simulink model "Helicopter_Interface"  (R2022a)
settings: Solver=ode1  StartTime=0.0  StopTime=inf  FixedStep=0.01  MaxStep=0.01  RelTol=1e-3
values from neighbouring files (symbols this model uses):
  A = eval(subs(A_,{x1,x2,x3,x4,x5,x6,F_f,F_b},{0,-5*pi/180,0,0,0,0, u_ap(1)   u_ap(2)}))    [solve.m]
  B = eval(subs(B_,{x1,x2,x3,x4,x5,x6,F_f,F_b},{0,-5*pi/180,0,0,0,0, u_ap(1)   u_ap(2)}))    [solve.m]
  C = [1 0 0 0 0 0 ... (first row only)    [solve.m]
  L = place(A',C',p_beo)'    [Beobachter.m]
  V = -pinv(C*inv(A-B*K)*B)    [Beobachter.m]
undefined symbols (not defined in the file or in its folder): GUIdisplay, K_lqi, u_a, x_init
libraries: vrlib x4, simulink_extras x3
settings Model: Creator=kilia  LastModifiedBy=Lyn
settings SolverCC: AlgebraicLoopSolver=TrustRegion
settings DebuggingCC: UnconnectedInputMsg=warning  UnconnectedOutputMsg=warning  UnconnectedLineMsg=warning
settings RTWCC: DLArmComputeVersion=19.05

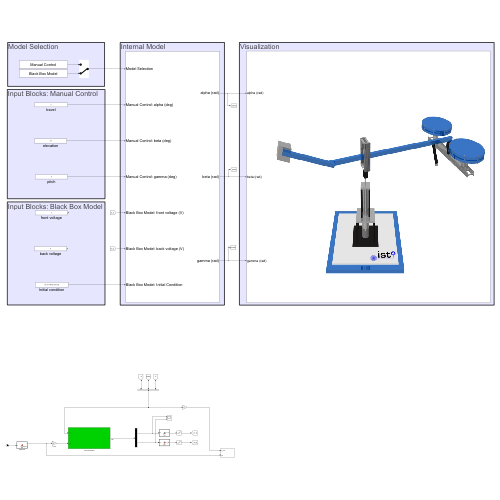
[thumbnail: Simulink's stored preview of the top-level diagram]
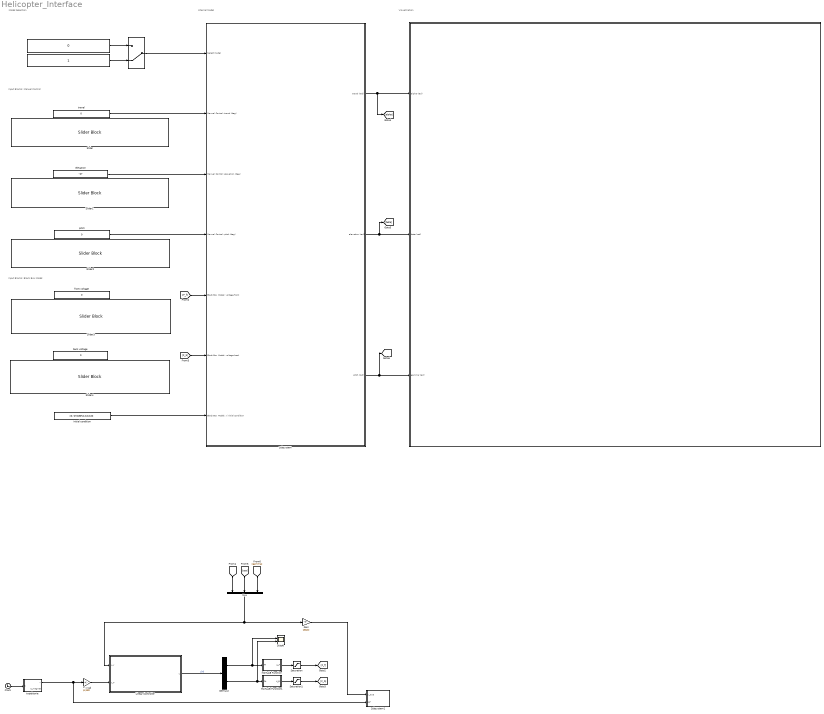
== system Helicopter_Interface ==
  note: Input Blocks: Black Box Model
  note: Internal Model
  note: Visualization
  note: Input Blocks: Manual Control
  note: Model Selection
  "  " : Subsystem
      mask Display: image('$imagefile'); % Use "Edit Image" on toolstrip to change.
  "   " : ManualSwitch  CurrentSetting=0
  "     " : Constant  Value=0
      mask Display: disp('Manual Control');
  "      " : Constant
      mask Display: disp('Black Box Model');
  Clock : Clock
  Demux2 : Demux  Outputs=2
  Gain : Gain  Gain=180/pi
  Initial condition : Constant  Value=[0,-27/180*pi,0,0,0,0]
  Linear Controller : Subsystem
  MATLAB Function : MATLAB Function  TreatAsAtomicUnit=on
  MATLAB Function1 : MATLAB Function  TreatAsAtomicUnit=on
  Mux : Mux  Inputs=3
  Saturation : Saturate  UpperLimit=4  LowerLimit=-4
  Saturation1 : Saturate  UpperLimit=4  LowerLimit=-4
  Scope : Scope  NumInputPorts=2
  Slider : SliderBlock  ScaleMin=-360  ScaleMax=360  TickInterval=90
  Slider1 : SliderBlock  ScaleMin=-27  ScaleMax=30
  Slider2 : SliderBlock  ScaleMin=-90  ScaleMax=90  TickInterval=15
  Slider3 : SliderBlock  ScaleMax=4  TickInterval=0.5
  Slider4 : SliderBlock  ScaleMax=4  TickInterval=0.5
  Subsystem : Subsystem
      mask Display:
      | port_label('input', 1, 'Model Selection');
      | port_label('input', 2, 'Manual Control: alpha (deg)');
      | port_label('input', 3, 'Manual Control: beta (deg)');
      | port_label('input', 4, 'Manual Control: gamma (deg)');
      | port_label('input', 5, 'Black Box Model: front voltage (V)');
      | port_label('input', 6, 'Black Box Model: back voltage (V)');
      | port_label('input', 7, 'Black Box Model: Initial Condition')
      | port_label('output', 1, 'alpha (rad)')
      | port_label('output', 2, 'beta (rad)')
      | port_label('output', 3, 'gamma (rad)')
  Subsystem1 : Subsystem
  back voltage : Constant  Value=0
  elevation : Constant  Value=-27
  front voltage : Constant  Value=0
  pitch : Constant  Value=0
  trajektorie : MATLAB Function  TreatAsAtomicUnit=on
  travel : Constant  Value=0
  °->rad : Gain  Gain=pi/180
  wires:
  "     "/1 -> "   "/1
  "      "/1 -> "   "/2
  "   "/1 -> Subsystem/1(Select model)
  travel/1 -> Subsystem/2(Manual Control: travel (deg))
  elevation/1 -> Subsystem/3(Manual Control: elevation (deg))
  pitch/1 -> Subsystem/4(Manual Control: pitch (deg))
  Initial condition/1 -> Subsystem/7(Black Box Model: x initial condition)
  Subsystem/1(travel (rad)) -> [alpha], "  "/1(alpha (rad))
  Subsystem/2(elevation (rad)) -> [beta], "  "/2(beta (rad))
  Subsystem/3(pitch (rad)) -> [gamma], "  "/3(gamma (rad))
  trajektorie/1(r) -> Subsystem1/2(ref), °->rad/1
  MATLAB Function1/1(U_B) -> Saturation1/1
  °->rad/1 -> Linear Controller/2(y_s)
  MATLAB Function/1(U_F) -> Saturation/1
  Linear Controller/1(u) -> Demux2/1  "u[N]"
  Clock/1 -> trajektorie/1(t)
  Demux2/1 -> Scope/1, MATLAB Function/1(Ff)
  Demux2/2 -> Scope/2, MATLAB Function1/1(Fb)
  Saturation/1 -> [F_f]
  Saturation1/1 -> [F_b]
  [F_f] -> Subsystem/5(Black Box Model: voltage front)
  [F_b] -> Subsystem/6(Black Box Model: voltage back)
  [alpha] -> Mux/1
  [beta] -> Mux/2
  [gamma] -> Mux/3
  Mux/1 -> Linear Controller/1(y_r), Gain/1
  Gain/1 -> Subsystem1/1(y_true)

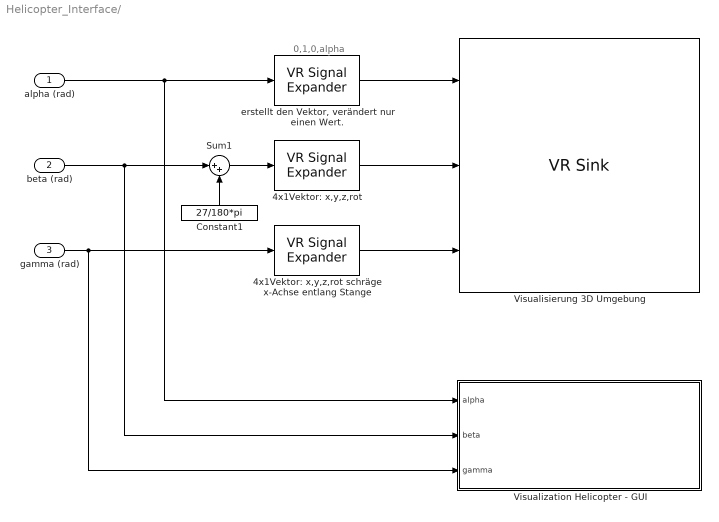
== system Helicopter_Interface/   ==
  note: 0,1,0,alpha
  alpha (rad) : Inport
  beta (rad) : Inport  Port=2
  gamma (rad) : Inport  Port=3
  4x1Vektor: x,y,z,rot : vrlib/VR Signal Expander  outwidth=4  outidx=[4]
  4x1Vektor: x,y,z,rot schräge x-Achse entlang Stange : vrlib/VR Signal Expander  outwidth=4  outidx=[4]
  Constant1 : Constant  Value=27/180*pi
  Sum1 : Sum  Inputs=|++
  Visualisierung 3D Umgebung : vrlib/VR Sink  InstantiateOnLoad=on  SampleTime=-1  ViewEnable=on  RemoteChange=off  RemoteView=off  FieldsWritten=Gelenk_alpha.rotation.4.1.1.double#Gelenk_beta.rotation.4.1.1.double#Gelenk_gamma.rotation.4.1.1.double  WorldFileName=ressources\VrWorld.x3d  AutoView=on  VideoDimensions=[]  AllowVariableSize=off  FigureProperties="{'Position', 'Name', 'Viewpoint', 'CameraBound', 'CameraDirection', 'CameraPosition', 'CameraUpVector', 'ZoomFactor', 'Antialiasing', 'Headlight', 'Lighting', 'NavPanel', 'Sound', 'StatusBar', 'Stereo3D', 'Stereo3DCameraOffset', 'Stereo3DHIT', 'ToolBar', 'Textures', 'Transparency', 'Triad', 'Wireframe', 'NavZones', 'NavMode', 'NavSpeed', 'CaptureFileFormat', 'CaptureFileName', 'Record2DCompressMethod', 'Record2DCompressQuality', 'Record2D', 'Record2DFileName', 'Record2DFPS'; [5.0000000000000000e+00   9.2000000000000000e+01   5.7600000000000000e+02   3.5000000000000000e+02], '', 'seitlich', 'on', [0.0000000000000000e+00   0.0000000000000000e+00  -1.0000000000000000e+00], [0.0000000000000000e+00   0.0000000000000000e+00   0.0000000000000000e+00], [0.0000000000000000e+00   1.0000000000000000e+00   0.0000000000000000e+00], [1.0000000000000000e+00], 'off', 'on', 'on', 'halfbar', 'on', 'on', 'off', [1.0000000149011612e-01], [0.0000000000000000e+00], 'on', 'on', 'on', 'none', 'off', 'off', 'fly', 'normal', 'tif', '%f_anim_%n.tif', 'auto', [7.5000000000000000e+01], 'off', '%f_anim_%n.avi', 'auto'}"
  Visualization Helicopter - GUI : Subsystem  LoadFcn=GUIdisplay([], [], [], 'LoadBlock', [], [])  StartFcn=GUIdisplay([], [], [], 'Start', [], 'ressources/VrWorld.x3d')  StopFcn=GUIdisplay([], [], [], 'Stop', [], [])  mask(Grafische Benutzeroberfläche){y1range=[-100 470], y2range=[-32 35], y3range=[-95 95], worldfile=ressources/VrWorld.x3d}
      mask prompts: y1range "Alpha range:"; y2range "Beta range:"; y3range "Gamma range:"; worldfile "VRML World Datei:"
      mask help:
      | Anzeige der grafischen Benutzeroberfläche.
      |
      | 2 VR Kameraperspektiven,
      | 3 Plots für die 3 Winkel.
      settings: CopyFcn=GUIdisplay([], [], [], 'CopyBlock', [], [])  DeleteFcn=GUIdisplay([], [], [], 'DeleteBlock', [], [])  NameChangeFcn=GUIdisplay([], [], [], 'NameChange', [], [])
      mask Display:
      | port_label('input',1,'alpha');
      | port_label('input',2,'beta');
      | port_label('input',3,'gamma');
      | image('ressources/GUImask.png');
  "erstellt den Vektor, verändert nur einen Wert." : vrlib/VR Signal Expander  outwidth=4  outidx=[4]
  wires:
  alpha (rad)/1 -> "erstellt den Vektor, verändert nur einen Wert."/1, Visualization Helicopter - GUI/1(alpha)
  "erstellt den Vektor, verändert nur einen Wert."/1 -> Visualisierung 3D Umgebung/1
  4x1Vektor: x,y,z,rot/1 -> Visualisierung 3D Umgebung/2
  4x1Vektor: x,y,z,rot schräge x-Achse entlang Stange/1 -> Visualisierung 3D Umgebung/3
  Constant1/1 -> Sum1/2
  beta (rad)/1 -> Sum1/1, Visualization Helicopter - GUI/2(beta)
  gamma (rad)/1 -> 4x1Vektor: x,y,z,rot schräge x-Achse entlang Stange/1, Visualization Helicopter - GUI/3(gamma)
  Sum1/1 -> 4x1Vektor: x,y,z,rot/1

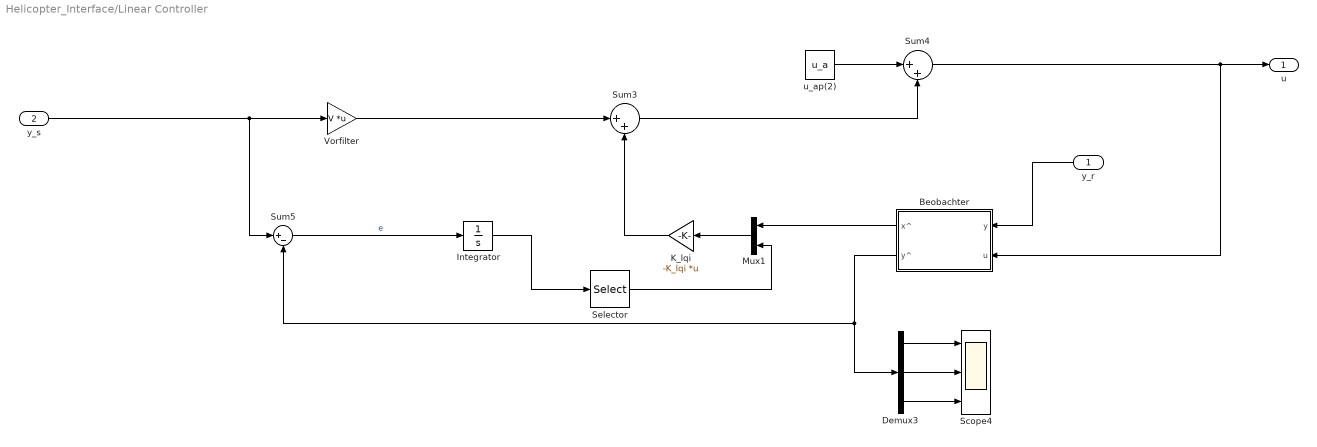
== system Helicopter_Interface/Linear Controller ==
  y_r : Inport
  y_s : Inport  Port=2
  Beobachter : Subsystem
  Demux3 : Demux  Outputs=3
  Integrator : Integrator
  K_lqi : Gain  Gain=-K_lqi  Multiplication=Matrix(K*u) (u vector)
  Mux1 : Mux  Inputs=2
  Scope4 : Scope  NumInputPorts=3
  Selector : Selector  InputPortWidth=3  IndexOptions=Index vector (dialog)  Indices=[1 2]  OutputSizes=1
  Sum3 : Sum  Inputs=|++
  Sum4 : Sum  Inputs=|++
  Sum5 : Sum  Inputs=|+-
  Vorfilter : Gain  Gain=V  Multiplication=Matrix(K*u) (u vector)
  u_ap(2) : Constant  Value=u_a  VectorParams1D=off
  u : Outport
  wires:
  u_ap(2)/1 -> Sum4/1
  Sum3/1 -> Sum4/2
  Sum5/1 -> Integrator/1  "e"
  Beobachter/1(x^) -> Mux1/1
  Demux3/2 -> Scope4/2
  K_lqi/1 -> Sum3/2
  Sum4/1 -> Beobachter/2(u), u/1
  Demux3/1 -> Scope4/1
  Mux1/1 -> K_lqi/1
  Vorfilter/1 -> Sum3/1
  y_s/1 -> Vorfilter/1, Sum5/1
  Beobachter/2(y^) -> Sum5/2, Demux3/1
  Integrator/1 -> Selector/1
  Selector/1 -> Mux1/2
  Demux3/3 -> Scope4/3
  y_r/1 -> Beobachter/1(y)

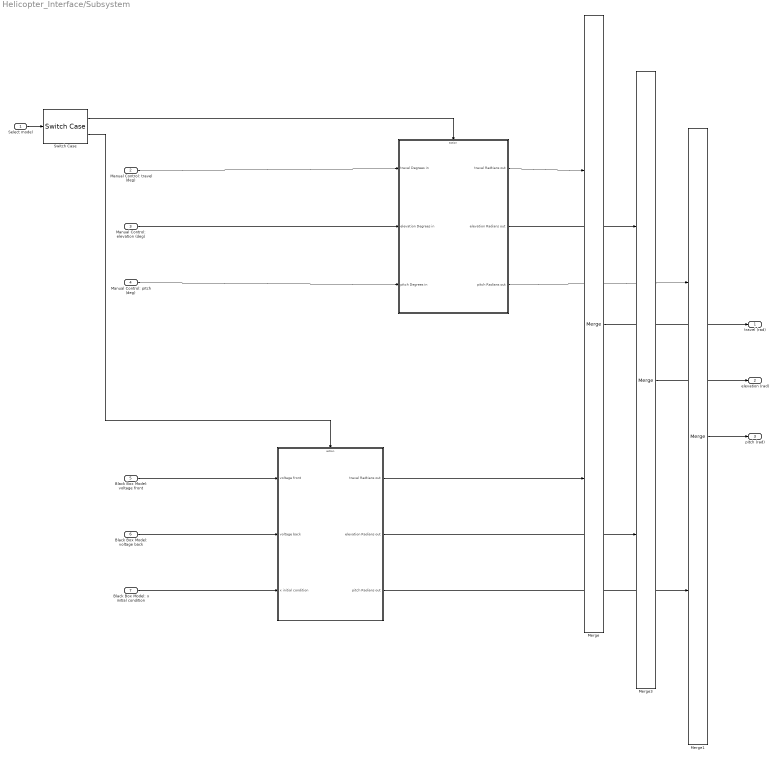
== system Helicopter_Interface/Subsystem ==
  Select model : Inport
  Manual Control: travel (deg) : Inport  Port=2
  Manual Control: elevation (deg) : Inport  Port=3
  Manual Control: pitch (deg) : Inport  Port=4
  Black Box Model: voltage front : Inport  Port=5
  Black Box Model: voltage back : Inport  Port=6
  Black Box Model: x initial condition : Inport  Port=7
  " " : Subsystem  TreatAsAtomicUnit=on
      mask Display: disp('Manual Control');
  "  " : Subsystem  TreatAsAtomicUnit=on
      mask Display: disp('Black Box Model');
  Merge : Merge
  Merge1 : Merge
  Merge3 : Merge
  Switch Case : SwitchCase  CaseConditions={0,1}  ShowDefaultCase=off
  travel (rad) : Outport
  elevation (rad) : Outport  Port=2
  pitch (rad) : Outport  Port=3
  wires:
  "  "/1(travel Radtians out) -> Merge/2
  " "/1(travel Radtians out) -> Merge/1
  "  "/2(elevation Radians out) -> Merge3/2
  Black Box Model: x initial condition/1 -> "  "/3(x initial condition)
  "  "/3(pitch Radians out) -> Merge1/2
  " "/3(pitch Radians out) -> Merge1/1
  " "/2(elevation Radians out) -> Merge3/1
  Switch Case/1 -> " "/Action
  Manual Control: elevation (deg)/1 -> " "/2(elevation Degrees in)
  Switch Case/2 -> "  "/Action
  Merge3/1 -> elevation (rad)/1
  Merge1/1 -> pitch (rad)/1
  Merge/1 -> travel (rad)/1
  Black Box Model: voltage back/1 -> "  "/2(voltage back)
  Manual Control: pitch (deg)/1 -> " "/3(pitch Degrees in)
  Black Box Model: voltage front/1 -> "  "/1(voltage front)
  Manual Control: travel (deg)/1 -> " "/1(travel Degrees in)
  Select model/1 -> Switch Case/1

== system Helicopter_Interface/Subsystem1 ==
  y_true : Inport
  ref : Inport  Port=2
  Demux : Demux  Outputs=3
  Demux1 : Demux  Outputs=3
  Scope : Subsystem
  wires:
  Demux/2 -> Scope/2(beta_r[°])  "beta_r[°]"
  Demux1/1 -> Scope/4(alpha_s[°])
  Demux1/3 -> Scope/6(gamma_s[°])
  Demux/3 -> Scope/3(gamma_r[°])
  Demux1/2 -> Scope/5(beta_s[°])
  Demux/1 -> Scope/1(alpha_r[°])  "alpha_r[°]"
  y_true/1 -> Demux/1
  ref/1 -> Demux1/1

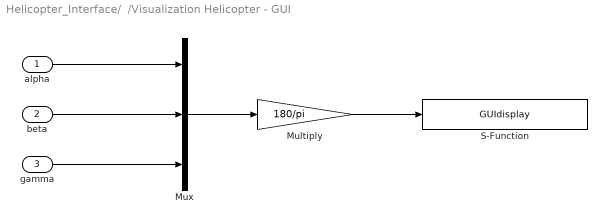
== system Helicopter_Interface/  /Visualization Helicopter - GUI ==
  alpha : Inport
  beta : Inport  Port=2
  gamma : Inport  Port=3
  Multiply : Gain  Gain=180/pi
  Mux : Mux  Inputs=3
  S-Function : S-Function  FunctionName=GUIdisplay  Parameters=[y1range y2range y3range], worldfile  SFunctionDeploymentMode=off  EnableBusSupport=off
  wires:
  Multiply/1 -> S-Function/1
  alpha/1 -> Mux/1
  gamma/1 -> Mux/3
  Mux/1 -> Multiply/1
  beta/1 -> Mux/2

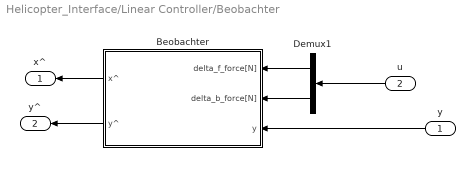
== system Helicopter_Interface/Linear Controller/Beobachter ==
  y : Inport
  u : Inport  Port=2
  Beobachter : Subsystem
  Demux1 : Demux  Outputs=2
  x^ : Outport
  y^ : Outport  Port=2
  wires:
  u/1 -> Demux1/1
  Demux1/1 -> Beobachter/1(delta_f_force[N])
  Demux1/2 -> Beobachter/2(delta_b_force[N])
  Beobachter/1(x^) -> x^/1
  y/1 -> Beobachter/3(y)
  Beobachter/2(y^) -> y^/1

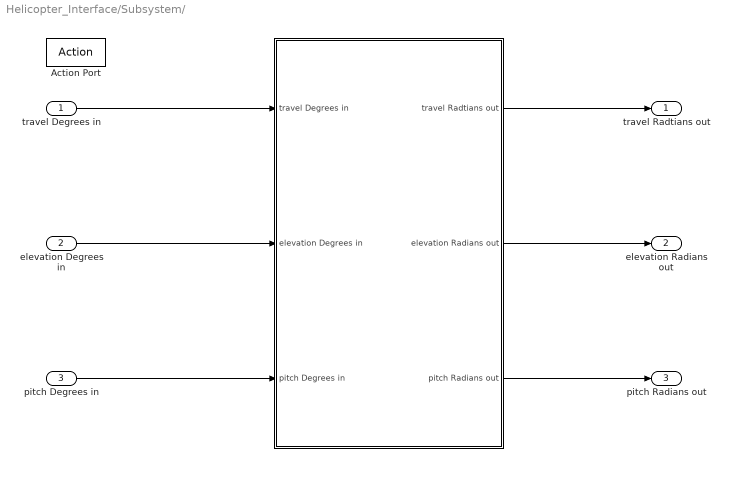
== system Helicopter_Interface/Subsystem/  ==
  travel Degrees in : Inport
  elevation Degrees in : Inport  Port=2
  pitch Degrees in : Inport  Port=3
  Action Port : ActionPort  ActionPortLabel=case [ 0 ]:
  " " : Subsystem
  travel Radtians out : Outport
  elevation Radians out : Outport  Port=2
  pitch Radians out : Outport  Port=3
  wires:
  " "/2(elevation Radians out) -> elevation Radians out/1
  " "/1(travel Radtians out) -> travel Radtians out/1
  " "/3(pitch Radians out) -> pitch Radians out/1
  travel Degrees in/1 -> " "/1(travel Degrees in)
  elevation Degrees in/1 -> " "/2(elevation Degrees in)
  pitch Degrees in/1 -> " "/3(pitch Degrees in)

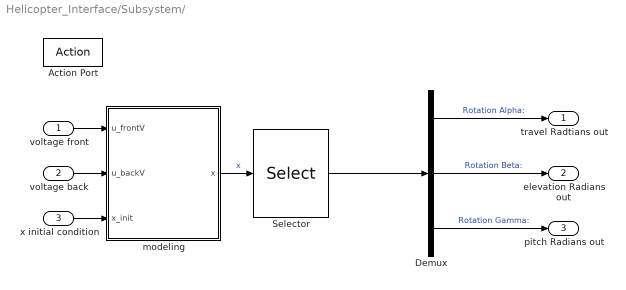
== system Helicopter_Interface/Subsystem/   ==
  voltage front : Inport
  voltage back : Inport  Port=2
  x initial condition : Inport  Port=3
  Action Port : ActionPort  ActionPortLabel=case [ 1 ]:
  Demux : Demux  Outputs=3
  Selector : Selector  InputPortWidth=6  IndexOptions=Index vector (dialog)  Indices=[1 2 3]  OutputSizes=1
  modeling : Subsystem
  travel Radtians out : Outport
  elevation Radians out : Outport  Port=2
  pitch Radians out : Outport  Port=3
  wires:
  Selector/1 -> Demux/1
  Demux/1 -> travel Radtians out/1  "Rotation Alpha:"
  modeling/1(x) -> Selector/1  "x"
  Demux/3 -> pitch Radians out/1  "Rotation Gamma:"
  Demux/2 -> elevation Radians out/1  "Rotation Beta:"
  voltage front/1 -> modeling/1(u_frontV)
  voltage back/1 -> modeling/2(u_backV)
  x initial condition/1 -> modeling/3(x_init)

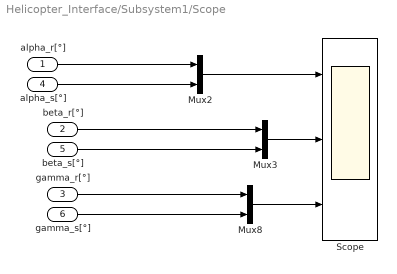
== system Helicopter_Interface/Subsystem1/Scope ==
  alpha_r[°] : Inport
  beta_r[°] : Inport  Port=2
  gamma_r[°] : Inport  Port=3
  alpha_s[°] : Inport  Port=4
  beta_s[°] : Inport  Port=5
  gamma_s[°] : Inport  Port=6
  Mux2 : Mux  Inputs=2
  Mux3 : Mux  Inputs=2
  Mux8 : Mux  Inputs=2
  Scope : Scope  NumInputPorts=3
  wires:
  Mux8/1 -> Scope/3
  Mux2/1 -> Scope/1
  Mux3/1 -> Scope/2
  gamma_r[°]/1 -> Mux8/1
  beta_r[°]/1 -> Mux3/1
  alpha_s[°]/1 -> Mux2/2
  alpha_r[°]/1 -> Mux2/1
  beta_s[°]/1 -> Mux3/2
  gamma_s[°]/1 -> Mux8/2

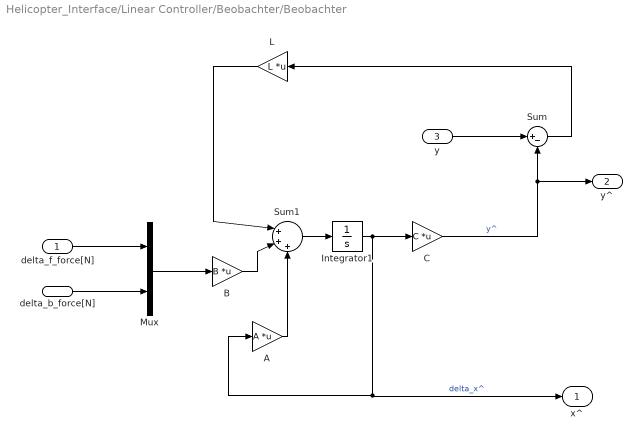
== system Helicopter_Interface/Linear Controller/Beobachter/Beobachter ==
  delta_f_force[N] : Inport
  delta_b_force[N] : Inport  Port=2
  y : Inport  Port=3
  A : Gain  Gain=A  Multiplication=Matrix(K*u) (u vector)
  B : Gain  Gain=B  Multiplication=Matrix(K*u) (u vector)
  C : Gain  Gain=C  Multiplication=Matrix(K*u) (u vector)
  Integrator1 : Integrator  InitialCondition=[0;-27*pi/180;0;0;0;0]
  L : Gain  Gain=L  Multiplication=Matrix(K*u) (u vector)
  Mux : Mux  Inputs=2
  Sum : Sum  Inputs=|+-
  Sum1 : Sum  Inputs=|+++
  x^ : Outport
  y^ : Outport  Port=2
  wires:
  Sum1/1 -> Integrator1/1
  Integrator1/1 -> C/1, x^/1, A/1  "delta_x^"
  B/1 -> Sum1/2
  L/1 -> Sum1/1
  Sum/1 -> L/1
  Mux/1 -> B/1
  A/1 -> Sum1/3
  C/1 -> y^/1, Sum/2  "y^"
  delta_f_force[N]/1 -> Mux/1
  delta_b_force[N]/1 -> Mux/2
  y/1 -> Sum/1

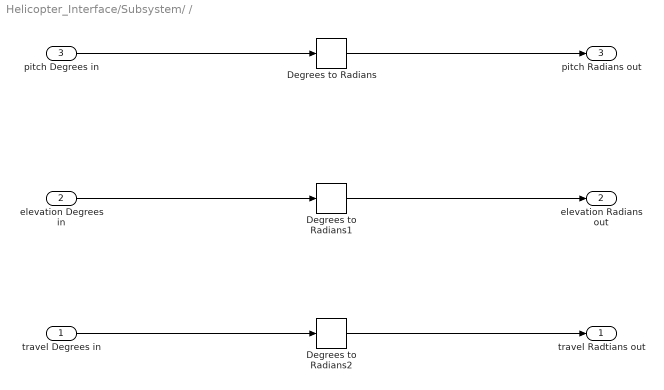
== system Helicopter_Interface/Subsystem/ /  ==
  travel Degrees in : Inport
  elevation Degrees in : Inport  Port=2
  pitch Degrees in : Inport  Port=3
  Degrees to Radians : simulink_extras/Transformations/Degrees to Radians
  Degrees to Radians1 : simulink_extras/Transformations/Degrees to Radians
  Degrees to Radians2 : simulink_extras/Transformations/Degrees to Radians
  travel Radtians out : Outport
  elevation Radians out : Outport  Port=2
  pitch Radians out : Outport  Port=3
  wires:
  pitch Degrees in/1 -> Degrees to Radians/1
  Degrees to Radians/1 -> pitch Radians out/1
  Degrees to Radians2/1 -> travel Radtians out/1
  Degrees to Radians1/1 -> elevation Radians out/1
  travel Degrees in/1 -> Degrees to Radians2/1
  elevation Degrees in/1 -> Degrees to Radians1/1

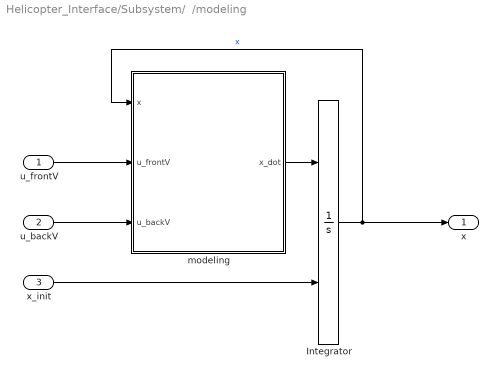
== system Helicopter_Interface/Subsystem/  /modeling ==
  u_frontV : Inport
  u_backV : Inport  Port=2
  x_init : Inport  Port=3
  Integrator : Integrator  InitialConditionSource=external  InitialCondition=x_init
  modeling : MATLAB Function  TreatAsAtomicUnit=on
  x : Outport
  wires:
  modeling/1(x_dot) -> Integrator/1
  Integrator/1 -> x/1, modeling/1(x)  "x"
  x_init/1 -> Integrator/2
  u_backV/1 -> modeling/3(u_backV)
  u_frontV/1 -> modeling/2(u_frontV)

== matlab function Helicopter_Interface/MATLAB Function ==
  data: Ff input; U_F output
function U_F = fcn(Ff)
    U_F= sqrt(20*abs(Ff));
end

== matlab function Helicopter_Interface/Subsystem/  /modeling/modeling ==
  data: x input; x_dot output; u_frontV input; u_backV input
function x_dot = modeling(x,u_frontV,u_backV)
    if u_frontV > 4
        u_frontV = 4;
    elseif u_frontV < -4
        u_frontV = -4;
    end
    if u_backV > 4
        u_backV = 4;
    elseif u_backV < -4
        u_backV = -4;
    end
    t2 = cos(x(2));
    t3 = cos(x(3));
    t4 = sin(x(2));
    t5 = sin(x(3));
    t6 = x(4).^2;
    t7 = x(2).*2.0;
    t8 = x(5).^2;
    t9 = x(3).*2.0;
    t10 = x(6).^2;
    t11 = u_backV.^2;
    t12 = u_frontV.^2;
    t48 = x(4).*x(5).*2.03058268355089e-1;
    t13 = cos(t7);
    t14 = t2.^2;
    t15 = t3.^2;
    t16 = t3.^3;
    t18 = sin(t7);
    t19 = t4.^2;
    t20 = sin(t9);
    t21 = t5.^2;
    t23 = t2.*t8.*1.635155998723047e-2;
    t25 = t11.*9.174434079640917e-3;
    t26 = t12.*9.174434079640917e-3;
    t27 = x(4).*x(5).*t2.*7.452385e-2;
    t28 = t4.*t8.*4.862799017853676e-4;
    t29 = x(4).*x(6).*t2.*7.452385e-2;
    t33 = t3.*t11.*3.385495392768902e-2;
    t34 = t3.*t12.*3.385495392768902e-2;
    t35 = t5.*t11.*2.946156295997365e-3;
    t36 = t5.*t12.*2.946156295997365e-3;
    t41 = t2.*t5.*t11.*3.385495392768902e-2;
    t42 = t2.*t5.*t12.*3.385495392768902e-2;
    t43 = t4.*t12.*(-9.174434079640917e-3);
    t44 = t4.*t5.*t11.*4.600138777960798e-3;
    t45 = t4.*t5.*t12.*4.600138777960798e-3;
    t46 = t2.*t3.*t11.*2.946156295997365e-3;
    t47 = t2.*t3.*t12.*2.946156295997365e-3;
    t49 = t6.*1.015291341775445e-1;
    t50 = -t48;
    t52 = x(4).*x(5).*t3.*2.774580000000001e-3;
    t53 = x(4).*x(6).*t5.*3.770040000000002e-4;
    t54 = x(5).*x(6).*t5.*3.770040000000002e-4;
    t55 = t3.*t6.*1.387290000000001e-3;
    t57 = t3.*t10.*1.387290000000001e-3;
    t58 = t5.*t6.*1.885020000000001e-4;
    t59 = t5.*t8.*1.885020000000001e-4;
    t64 = x(4).*x(6).*t3.*t4.*2.774580000000001e-3;
    t65 = x(4).*x(5).*t2.*t3.*3.770040000000002e-4;
    t66 = x(4).*x(6).*t2.*t3.*3.770040000000002e-4;
    t68 = x(4).*x(5).*t2.*t3.*t4.*7.540080000000003e-4;
    t69 = t2.*t5.*t8.*1.387290000000001e-3;
    t70 = x(4).*x(5).*t3.*t4.*(-2.774580000000001e-3);
    t71 = t2.*t5.*t10.*1.387290000000001e-3;
    t74 = t4.*t5.*t10.*1.885020000000001e-4;
    t75 = x(4).*x(6).*t2.*t4.*t5.*2.774580000000001e-3;
    t80 = t2.*t4.*t5.*t6.*1.387290000000001e-3;
    t82 = t2.*t3.*t4.*t6.*3.770040000000002e-4;
    t91 = t2.*8.248718165204683e-1;
    t92 = t2.*t5.*4.155516000000001e-2;
    t93 = t3.*t4.*4.155516000000001e-2;
    t94 = t4.*1.324177010693453;
    t95 = t2.*6.321561677527197e+77;
    t97 = t3.*1.225248066969451e+78;
    t98 = t2.*t5.*2.450496133938901e+77;
    t99 = t4.*2.125676891098147e+79;
    t100 = t2.*t5.*7.094850583348527e+78;
    t101 = t3.*t5.*1.100101830038337e+78;
    t102 = x(5).*x(6).*t2.*2.73147057186082e-3;
    t103 = t3.*t4.*t5.*8.800814640306698e+75;
    t105 = t5.*3.48026202342401e+81;
    t106 = t2.*t3.*t5.*6.477004033034705e+76;
    t107 = t4.*t5.*2.385701619337445e+80;
    t112 = t2.*t4.*7.901952096908996e+79;
    t113 = t3.*t4.*2.509206552712654e+81;
    t114 = t4.*4.827997583224782e+83;
    t119 = t2.*t4.*t5.*3.063120167423627e+79;
    t132 = t2.*t3.*t4.*9.50424515204181e+79;
    t133 = t2.*t3.*1.733947310723218e+82;
    t146 = t2.*t3.*t4.*t5.*7.946775555990462e+78;
    t158 = t3.*t4.*t5.*t8.*3.589618971406959e-2;
    t171 = t3.*9.694963676602881e+122;
    t174 = t2.*t4.*3.434970881571123e+121;
    t187 = t2.*t4.*t5.*1.331535353899349e+121;
    t193 = t2.*t3.*t4.*t5.*3.505212574967064e+120;
    t223 = t2.*t3.*t4.*7.122357460232167e+123;
    t17 = t15.^2;
    t22 = t20.^2;
    t24 = -t23;
    t30 = -t26;
    t31 = -t28;
    t32 = -t29;
    t37 = -t33;
    t38 = -t34;
    t39 = t4.*t25;
    t40 = t4.*t26;
    t51 = x(4).*x(5).*t14.*4.061165367101779e-1;
    t56 = -t52;
    t60 = -t53;
    t61 = -t54;
    t62 = t6.*t14.*2.03058268355089e-1;
    t63 = t4.*t52;
    t72 = -t66;
    t73 = t4.*t59;
    t76 = -t71;
    t77 = -t74;
    t78 = x(4).*x(5).*t3.*t14.*5.549160000000002e-3;
    t79 = t14.*t53;
    t81 = -t75;
    t83 = t3.*t6.*t14.*2.774580000000001e-3;
    t84 = t14.*t58;
    t85 = -t82;
    t86 = x(4).*x(5).*t18.*1.086802113522521;
    t88 = t5.*t6.*t14.*(-1.885020000000001e-4);
    t89 = t6.*t18.*5.434010567612607e-1;
    t96 = -t95;
    t104 = -t100;
    t108 = t2.*t15.*5.500509150191686e+78;
    t109 = t3.*t14.*2.837940233339411e+78;
    t110 = t2.*t21.*2.750254575095843e+78;
    t111 = t15.*1.166611947319722e+80;
    t116 = t3.*t19.*1.296656147304016e+79;
    t117 = t4.*t21.*2.024063760323345e+79;
    t118 = t19.*2.657096113872683e+81;
    t120 = t2.*t20.*2.333223894639443e+79;
    t121 = -t112;
    t122 = t13.*t101;
    t123 = t14.*t101;
    t124 = t19.*t101;
    t125 = t2.*t16.*5.237273874528027e+80;
    t126 = t4.*t16.*7.116295798977013e+79;
    t127 = t5.*t15.*1.047454774905605e+80;
    t128 = t5.*t18.*5.925262666227655e+80;
    t130 = t5.*t19.*2.254318774901658e+80;
    t131 = x(5).*x(6).*t20.*3.589618971406959e-2;
    t135 = t3.*t5.*t13.*-1.100101830038337e+78;
    t136 = t3.*t5.*t18.*8.096255041293381e+78;
    t137 = t3.*t5.*t19.*-1.100101830038337e+78;
    t139 = x(4).*x(5).*t2.*t15.*7.179237942813918e-2;
    t140 = x(4).*x(6).*t2.*t15.*7.179237942813918e-2;
    t141 = x(5).*x(6).*t2.*t15.*7.179237942813918e-2;
    t142 = t5.*t13.*3.171300553775711e+81;
    t145 = t8.*t20.*1.79480948570348e-2;
    t147 = t2.*t5.*t20.*2.618636937264013e+80;
    t150 = -t146;
    t151 = t4.*t15.*1.458190194407001e+82;
    t152 = t2.*t3.*t4.*t20.*1.423259159795403e+79;
    t154 = x(4).*x(6).*t3.*t5.*t14.*7.179237942813918e-2;
    t156 = t2.*t4.*t20.*2.916529868299304e+81;
    t160 = x(4).*x(5).*t2.*t4.*t15.*(-7.179237942813918e-2);
    t164 = t3.*t14.*t20.*1.047454774905605e+80;
    t165 = -t158;
    t166 = t2.*t4.*t6.*t15.*3.589618971406959e-2;
    t167 = t3.*t5.*t6.*t14.*3.589618971406959e-2;
    t169 = t14.*5.107638978270105e+119;
    t170 = t3.*t21.*2.028614954006237e+118;
    t172 = t5.*t14.*3.959859986591955e+119;
    t173 = t21.*6.417689155495646e+121;
    t175 = -t171;
    t177 = t15.*1.641540254081147e+122;
    t178 = t14.*t16.*4.057229908012474e+118;
    t179 = t14.*t21.*7.675019309373171e+118;
    t181 = -t174;
    t182 = t3.*t5.*t14.*1.046646381040499e+119;
    t183 = t3.*t5.*t19.*4.782131942337327e+119;
    t184 = t3.*t13.*4.138462702746391e+121;
    t191 = t3.*t14.*t21.*4.057229908012474e+118;
    t192 = t3.*t19.*t21.*4.057229908012474e+118;
    t195 = t15.*t21.*1.931532483628991e+120;
    t196 = t19.*t21.*4.157019516732514e+120;
    t197 = t2.*t3.*t4.*t21.*2.93081009208969e+119;
    t198 = t2.*t4.*t15.*3.7016311010743e+121;
    t200 = t3.*t18.*3.643855631716766e+123;
    t201 = t3.*t19.*9.992258694036609e+122;
    t202 = t3.*t13.*t21.*-2.028614954006237e+118;
    t203 = t18.*2.606256753239576e+125;
    t204 = t19.*9.973487007685766e+124;
    t205 = t3.*t18.*t21.*1.492969432442792e+119;
    t207 = t13.*t16.*2.923087810085905e+121;
    t209 = t13.*t21.*5.847956572177934e+121;
    t210 = t14.*t20.*3.770354832305701e+121;
    t211 = t16.*t19.*2.923012902287755e+121;
    t212 = t18.*t21.*1.09263307476776e+121;
    t215 = t2.*t4.*t16.*2.151150995944596e+122;
    t217 = t13.*1.394912588759959e+126;
    t220 = t14.*t15.*1.27897667213932e+122;
    t221 = t16.*t18.*1.075630626745094e+122;
    t225 = t2.*t4.*t20.*1.267812693620274e+123;
    t227 = t5.*t14.*t20.*1.461543905042952e+121;
    t228 = t13.*t15.*3.940256742008736e+123;
    t230 = t15.*t19.*2.992314274899525e+123;
    t231 = t2.*t3.*t4.*t5.*t20.*5.249050108182602e+119;
    t233 = t3.*t5.*t14.*t20.*3.863064967257982e+120;
    t237 = t15.*t18.*7.870897512302404e+123;
    t67 = -t62;
    t87 = -t83;
    t90 = -t86;
    t115 = -t109;
    t129 = -t117;
    t134 = -t120;
    t138 = -t125;
    t143 = -t126;
    t144 = -t130;
    t148 = -t139;
    t149 = -t145;
    t153 = t4.*t139;
    t155 = -t147;
    t157 = -t151;
    t159 = -t152;
    t161 = -t154;
    t162 = -t156;
    t163 = t13.*t127;
    t168 = -t164;
    t176 = -t172;
    t180 = t17.*t19.*7.132297093561092e+118;
    t185 = t17.*1.391599486765761e+123;
    t188 = t2.*t4.*t17.*1.04981002163652e+120;
    t189 = -t182;
    t190 = t13.*t170;
    t194 = t14.*t17.*3.863064967257982e+120;
    t206 = -t192;
    t213 = -t196;
    t214 = -t197;
    t216 = -t200;
    t218 = -t203;
    t219 = -t207;
    t222 = -t211;
    t224 = -t215;
    t226 = -t217;
    t232 = -t225;
    t234 = -t227;
    t235 = -t228;
    t236 = -t230;
    t238 = -t231;
    t239 = t13.*t195;
    t240 = -t233;
    t241 = t14.*t22.*6.957997433828807e+122;
    t186 = -t180;
    t199 = -t188;
    t208 = -t194;
    t229 = t13.*t185;
    t242 = t96+t98+t99+t103+t106+t134;
    t243 = t25+t27+t30+t58+t59+t65+t70+t80+t88+t92+t148+t149+t167;
    t244 = t104+t107+t108+t110+t113+t114+t129+t133+t138+t143+t155+t157;
    t245 = t32+t35+t36+t37+t38+t49+t55+t57+t61+t64+t67+t72+t85+t87+t89+t91+t93+t94+t131+t140+t166;
    t246 = t24+t31+t39+t41+t42+t43+t44+t45+t46+t47+t50+t51+t56+t60+t68+t69+t73+t76+t77+t78+t79+t81+t90+t102+t141+t160+t161+t165;
    t247 = t101+t105+t115+t116+t118+t119+t121+t123+t127+t128+t132+t135+t136+t137+t142+t144+t150+t159+t162+t163+t168;
    t248 = t169+t170+t173+t175+t176+t177+t178+t179+t181+t183+t184+t185+t186+t187+t189+t191+t193+t195+t198+t199+t201+t202+t204+t205+t206+t208+t209+t210+t212+t213+t214+t216+t218+t219+t220+t221+t222+t223+t224+t226+t229+t232+t234+t235+t236+t237+t238+t239+t240+t241-1.530810853886889e+126;
    t249 = 1.0./t248;
    x_dot = [x(4);x(5);x(6);t242.*t245.*t249.*1.661534994731145e+45-t243.*t244.*t249.*5.316911983139663e+42-t246.*t249.*(t21.*1.619251008258676e+77-t97+t111-3.862398066579826e+81).*6.646139978924579e+44;t245.*t249.*(t13.*3.532063820998669e+81+t18.*6.599313290687543e+80-t19.*2.510767317953594e+80+t97+t111-t3.*t13.*1.225248066969451e+78+t3.*t18.*9.017275099606632e+78-t3.*t19.*2.450496133938901e+78-t14.*t15.*3.238502016517352e+77-t15.*t19.*5.979179412116765e+75+t13.*t111-t2.*t3.*t4.*1.803455019921326e+79-t2.*t4.*t15.*8.800814640306698e+76+3.876172369060467e+81).*3.32306998946229e+44+t242.*t246.*t249.*1.661534994731145e+45-t243.*t247.*t249.*1.329227995784916e+43;t244.*t246.*t249.*-5.316911983139663e+42-t245.*t247.*t249.*1.329227995784916e+43-t243.*t249.*(t3.*-4.95652853788659e+85-t13.*7.131459471819949e+88+t14.*2.611269026011294e+82+t15.*8.392337905379119e+84+t17.*7.114521311831996e+85-t18.*1.332442947224953e+88+t19.*2.952550677741535e+85-t2.*t4.*1.756121195420763e+84+t3.*t13.*2.115779818612926e+84-t5.*t14.*2.024469578668458e+82-t3.*t18.*1.862913057645561e+86-t5.*t19.*5.009973400608635e+84-t13.*t15.*2.014447463635022e+86-t13.*t16.*1.494422117785173e+84+t13.*t17.*7.114521311831996e+85+t15.*t18.*4.02397878319616e+86+t14.*t20.*1.927585491566282e+84+t16.*t18.*5.499137568254428e+84+t14.*t21.*3.923836489201627e+81+t14.*t22.*3.557260655915998e+85+t19.*t21.*2.125266948339513e+83+t2.*t4.*t5.*8.297363395849275e+83-t2.*t4.*t20.*6.48166409513115e+85-t2.*t4.*t21.*5.775534607701271e+82-t5.*t14.*t20.*7.472110588925864e+83+t2.*t4.*t5.*t20.*5.499137568254428e+84-7.826236318665165e+88).*5.063725698228251e+38];
end

== matlab function Helicopter_Interface/MATLAB Function1 ==
  data: Fb input; U_B output
function U_B = fcn(Fb)
    U_B= sqrt(20*abs(Fb));
end

== matlab function Helicopter_Interface/trajektorie ==
  data: t input; r output; U_magnet output
function [r, U_magnet] = fcn(t)
beta = -27;
if t <= 10
    a0 = five_times_plan(0, -27, 0, 0, 10, -5, 0, 0);
    alpha = 0;
    beta = a0(1)+a0(2)*t+a0(3)*t^2+a0(4)*t^3+a0(5)*t^4+a0(6)*t^5;
    U_magnet = 0;
elseif t > 10 && t <= 18
    a0 = five_times_plan(10, 0, 0, 0, 18, 90, 0, 0);
    alpha = a0(1)+a0(2)*t+a0(3)*t^2+a0(4)*t^3+a0(5)*t^4+a0(6)*t^5;
    beta = -5;
    U_magnet = 0;
elseif t > 18 &&t <= 26
    a0 = five_times_plan(18, -5, 0, 0, 26, -22, 0, 0);
    alpha = 90;
    beta = a0(1)+a0(2)*t+a0(3)*t^2+a0(4)*t^3+a0(5)*t^4+a0(6)*t^5;
    U_magnet = 1;
elseif t > 26 && t <= 30
    alpha = 90;
    beta = -22;
    U_magnet = 0;
elseif t > 30 && t <= 38
    a0 = five_times_plan(30, -22, 0, 0, 38, -5, 0, 0);
    alpha = 90;
    beta = a0(1)+a0(2)*t+a0(3)*t^2+a0(4)*t^3+a0(5)*t^4+a0(6)*t^5;
    U_magnet = 0;
elseif t > 38 && t <= 62
    a0 = five_times_plan(38, 90, 0, 0,62, 450, 0, 0);
    alpha = a0(1)+a0(2)*t+a0(3)*t^2+a0(4)*t^3+a0(5)*t^4+a0(6)*t^5;
    beta = -5;
    U_magnet = 0;
elseif t > 62 && t <= 70
    a0 = five_times_plan(62, -5, 0, 0, 70, -22, 0, 0); 
    alpha = 450;
    beta = a0(1)+a0(2)*t+a0(3)*t^2+a0(4)*t^3+a0(5)*t^4+a0(6)*t^5;
    U_magnet = 1;
elseif t > 70 && t <= 74
    alpha = 450;
    beta = -22;
    U_magnet = 0;
elseif t > 74 && t <= 82
    a0 = five_times_plan(74, -22, 0, 0, 82, -5, 0, 0);
    alpha = 450;
    beta = a0(1)+a0(2)*t+a0(3)*t^2+a0(4)*t^3+a0(5)*t^4+a0(6)*t^5;
    U_magnet = 0;
elseif t > 82 && t <= 110
    a0 = five_times_plan(82, 450, 0, 0, 110, 0, 0, 0);
    alpha = a0(1)+a0(2)*t+a0(3)*t^2+a0(4)*t^3+a0(5)*t^4+a0(6)*t^5;
    beta = -5;
    U_magnet = 0;
elseif t > 110 && t < 118
    a0 = five_times_plan(110, -5, 0, 0, 118, -27, 0, 0);
    alpha = 0;
    beta = a0(1)+a0(2)*t+a0(3)*t^2+a0(4)*t^3+a0(5)*t^4+a0(6)*t^5;
    U_magnet = 1;
else 
    alpha = 0; beta = -27;
    U_magnet = 0;
end
r = [alpha; beta;0];
function a = five_times_plan(ts, xs, vs, as, te, xe, ve, ae)
    para = [xs;vs;as;xe;ve;ae];
    Tran = [1,   ts,  ts^2,  ts^3,    ts^4,     ts^5;
            0,   1,   2*ts,  3*ts^2,  4*ts^3,   5*ts^4;
            0,   0,   2,     6*ts,    12*ts^2,  20*ts^3;
            1,   te,  te^2,  te^3,    te^4,     te^5;
            0,   1,   2*te,  3*te^2,  4*te^3,   5*te^4;
            0,   0,   2,     6*te,    12*te^2,  20*te^3];
    a = inv(Tran)*para;
end
end
